simulink model "DCM"  (R2020b)
settings: Solver=ode4  StartTime=0.0  StopTime=SIMULPARAM.T_end  FixedStep=SIMULPARAM.Ts  RelTol=1e-3  EnableMultiTasking=on
undefined symbols (not defined in the file): BAT, C_current, C_speed, CHAS, Chopper, CYCL, DCM, ENV, TRANS
libraries: simulink x1
settings Model: Creator=Huy  LastModifiedBy=mikesimard
settings DataIOCC: SaveFormat=Array  SignalLoggingSaveFormat=ModelDataLogs  SaveOutput=off  SignalLogging=off  SaveTime=off  ReturnWorkspaceOutputs=off
settings OptimizationCC: ExpressionDepthLimit=2147483647  LifeSpan=inf
settings DebuggingCC: AlgebraicLoopMsg=none  SaveWithDisabledLinksMsg=none  UnderspecifiedInitializationDetection=Classic  MergeDetectMultiDrivingBlocksExec=none  MaxConsecutiveZCsMsg=none  SolverPrmCheckMsg=warning  FcnCallInpInsideContextMsg=warning  ModelReferenceDataLoggingMessage=none  ModelReferenceExtraNoncontSigs=none  StateNameClashWarn=warning  SFUnexpectedBacktrackingDiag=warning  SFNoUnconditionalDefaultTransitionDiag=warning  SFExecutionAtInitializationDiag=none  ArithmeticOperatorsInVariantConditions=warning
settings HardwareCC: ProdBitPerPointer=32  ProdBitPerSizeT=32  ProdBitPerPtrDiffT=32  ProdLargestAtomicFloat=None  ProdIntDivRoundTo=Undefined  ProdEndianess=Unspecified  ProdWordSize=32  ProdHWDeviceType=32-bit Generic
settings ModelReferenceCC: PropagateSignalLabelsOutOfModel=off
settings SFSimCC: SimUseLocalCustomCode=off  CustomCodeUndefinedFunction=UseInterfaceOnly
settings RTWCC: RTWUseLocalCustomCode=off
settings CodeAppCC: StateflowObjectComments=on
settings GRTTargetCC: TargetLangStandard=C89/C90 (ANSI)  CombineOutputUpdateFcns=off  GRTInterface=on
settings ConfigComp: CovMetricSettings=dw  CovSaveCumulativeToWorkspaceVar=on  CovSaveSingleToWorkspaceVar=on  CovExternalEMLEnable=off

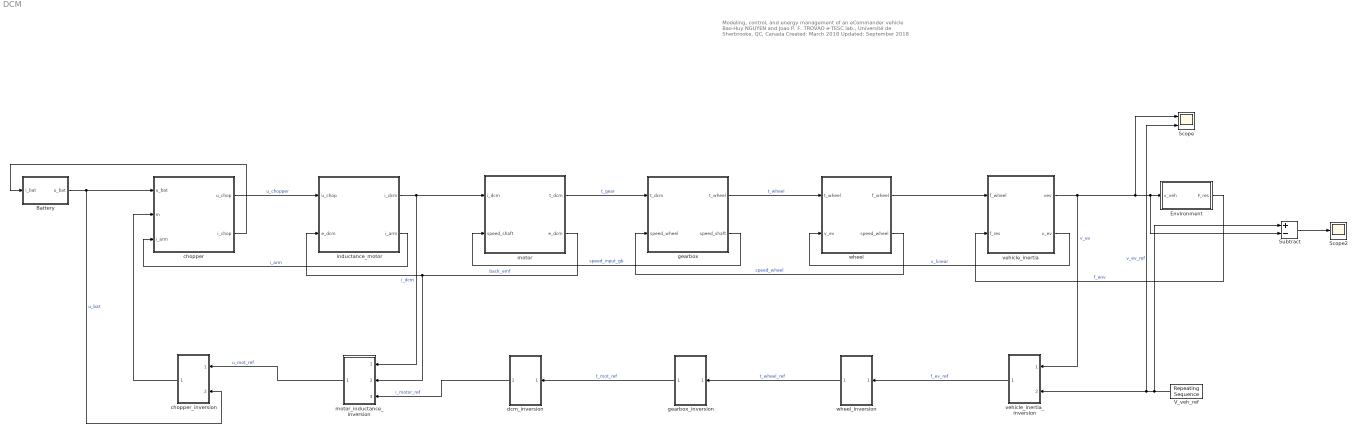
== system DCM ==
  note: Modeling, control, and energy management of an eCommander vehicle
      | Bao-Huy NGUYEN and Joao P. F. TROVAO
      | e-TESC lab., Université de Sherbrooke, QC, Canada
      | Created: March 2018        Updated: September 2018
  Battery : Subsystem  AncestorBlock=simulink/REM/SE
      mask Display:
      | plot(0,0,100,100, 1.2*[50,57.68,60.77,63.08,64.97,66.58,68,69.26,70.4, 	71.42,72.36,78.28,80,78.28,72.36,71.42,70.4, 	69.26,68,66.58,64.97,63.08,60.77,57.68,50,42.32, 	39.23,36.92,35.03,33.42,32,30.74,29.6,28.58, 	27.64,21.72,20,21.72,27.64,28.58,29.6,30.74,32, 	33.42,35.03,36.92,39.23,42.32,50]-10, 1.2*[20,21,22,23,24,25,26,27,28,29,30,40,50,60,70,71,72, 	73,74,75,76,77,78,79,80,79,78,77,76,75,74,73,72, 	71,70,60,50,40,30,29,28,27,26,25,24,23,22,21,20]-10)
      | disp('ES')
  Environment : Subsystem  AncestorBlock=simulink/REM/SE
      mask Display:
      | plot(0,0,100,100, 1.2*[50,57.68,60.77,63.08,64.97,66.58,68,69.26,70.4, 	71.42,72.36,78.28,80,78.28,72.36,71.42,70.4, 	69.26,68,66.58,64.97,63.08,60.77,57.68,50,42.32, 	39.23,36.92,35.03,33.42,32,30.74,29.6,28.58, 	27.64,21.72,20,21.72,27.64,28.58,29.6,30.74,32, 	33.42,35.03,36.92,39.23,42.32,50]-10, 1.2*[20,21,22,23,24,25,26,27,28,29,30,40,50,60,70,71,72, 	73,74,75,76,77,78,79,80,79,78,77,76,75,74,73,72, 	71,70,60,50,40,30,29,28,27,26,25,24,23,22,21,20]-10)
      | disp('MS')
  Scope : Scope  NumInputPorts=2
  Scope2 : Scope
  Subtract : Sum  Inputs=+-
  V_veh_ref : simulink/Sources/Repeating Sequence  rep_seq_t=CYCL.time  rep_seq_y=CYCL.velocity/1.25
  chopper : Subsystem  AncestorBlock=simulink/REM/EA  mask(CM){}
      mask Display: plot(0,0,100,100,[10,10,90,90,10],[90,10,10,90,90])
  chopper_inversion : Subsystem  AncestorBlock=simulink/SMC/Inversion EC avec mesure
      mask Display: plot(0,0,100,100,[10,30,90,70,10],[90,10,10,90,90])
  dcm_inversion : Subsystem  AncestorBlock=simulink/SMC/Inversion EC avec mesure
      mask Display: plot(0,0,100,100,[10,30,90,70,10],[90,10,10,90,90])
  gearbox : Subsystem  AncestorBlock=simulink/REM/EA  mask(CM){}
      mask Display: plot(0,0,100,100,[10,10,90,90,10],[90,10,10,90,90])
  gearbox_inversion : Subsystem  AncestorBlock=simulink/SMC/Inversion EC avec mesure
      mask Display: plot(0,0,100,100,[10,30,90,70,10],[90,10,10,90,90])
  inductance_motor : Subsystem  AncestorBlock=simulink/REM/EA  mask(CM){}
      mask Display: plot(0,0,100,100,[10,10,90,90,10],[90,10,10,90,90], [10,90],[10,90])
  motor : Subsystem  AncestorBlock=simulink/REM/EC EM
      mask Display: plot(0,0,100,100, 1.4*[50,57.68,60.77,63.08,64.97,66.58,68,69.26,70.4, 	71.42,72.36,78.28,80,78.28,72.36,71.42,70.4, 	69.26,68,66.58,64.97,63.08,60.77,57.68,50,42.32, 	39.23,36.92,35.03,33.42,32,30.74,29.6,28.58, 	27.64,21.72,20,21.72,27.64,28.58,29.6,30.74,32, 	33.42,35.03,36.92,39.23,42.32,50]-20, 1.4*[20,21,22,23,24,25,26,27,28,29,30,40,50,60,70,71,72, 	73,74,75,76,77,78,79,80,79,78,77,76,75,74,73,72, 	71,70,60,50,40,30,29,28,27,26,25,24,23,22,21,20]-20)
  motor_inductance_inversion : Subsystem  AncestorBlock=simulink/SMC/Asservissement Correcteur IP
      mask Display: plot(0,0,100,100, [10,30,90,70,10,90],[90,10,10,90,90,10])
  vehicle_inertia : Subsystem  AncestorBlock=simulink/REM/EA  mask(CM){}
      mask Display: plot(0,0,100,100,[10,10,90,90,10],[90,10,10,90,90], [10,90],[10,90])
  vehicle_inertia_inversion : Subsystem  AncestorBlock=simulink/SMC/Asservissement Correcteur IP
      mask Display: plot(0,0,100,100, [10,30,90,70,10,90],[90,10,10,90,90,10])
  wheel : Subsystem  AncestorBlock=simulink/REM/EA  mask(CM){}
      mask Display: plot(0,0,100,100,[10,10,90,90,10],[90,10,10,90,90])
  wheel_inversion : Subsystem  AncestorBlock=simulink/SMC/Inversion EC avec mesure
      mask Display: plot(0,0,100,100,[10,30,90,70,10],[90,10,10,90,90])
  wires:
  chopper_inversion/1(m_chopper) -> chopper/2(m)
  Battery/1(u_bat) -> chopper_inversion/2(u_bat), chopper/1(u_bat)  "u_bat"
  chopper/1(u_chop) -> inductance_motor/1(u_chop)  "u_chopper"
  vehicle_inertia/1(vev) -> Subtract/2, Environment/1(v_veh), Scope/1, vehicle_inertia_inversion/1(v_vehicle)  "v_ev"
  wheel/1(f_wheel) -> vehicle_inertia/1(f_wheel)
  inductance_motor/1(i_dcm) -> motor/1(i_dcm), motor_inductance_inversion/1(i_dcm)  "i_dcm"
  wheel/2(speed_wheel) -> gearbox/2(speed_wheel)  "speed_wheel"
  motor/2(e_dcm) -> inductance_motor/2(e_dcm), motor_inductance_inversion/2(back_emf)  "back_emf"
  motor/1(t_dcm) -> gearbox/1(t_dcm)  "t_gear"
  Environment/1(F_res) -> vehicle_inertia/2(f_res)  "f_env"
  inductance_motor/2(i_arm) -> chopper/3(i_arm)  "i_arm"
  gearbox/1(t_wheel) -> wheel/1(t_wheel)  "t_wheel"
  chopper/2(i_chop) -> Battery/1(i_bat)
  gearbox/2(speed_shaft) -> motor/2(speed_shaft)  "speed_input_gb"
  vehicle_inertia/2(v_ev) -> wheel/2(v_ev)  "v_linear"
  V_veh_ref/1 -> Subtract/1, Scope/2, vehicle_inertia_inversion/2(v_vehicle_ref)  "v_ev_ref"
  vehicle_inertia_inversion/1(f_vehicle_ref) -> wheel_inversion/1(f_vehicle_ref)  "f_ev_ref"
  wheel_inversion/1(t_wheel_ref) -> gearbox_inversion/1(t_wheel_ref)  "t_wheel_ref"
  gearbox_inversion/1(t_motor_ref) -> dcm_inversion/1(t_motor_ref)  "t_mot_ref"
  dcm_inversion/1(i_motor_ref) -> motor_inductance_inversion/3(i_motor_ref)  "i_motor_ref"
  motor_inductance_inversion/1(u_mot_ref) -> chopper_inversion/1(u_mot_ref)  "u_mot_ref"
  Subtract/1 -> Scope2/1

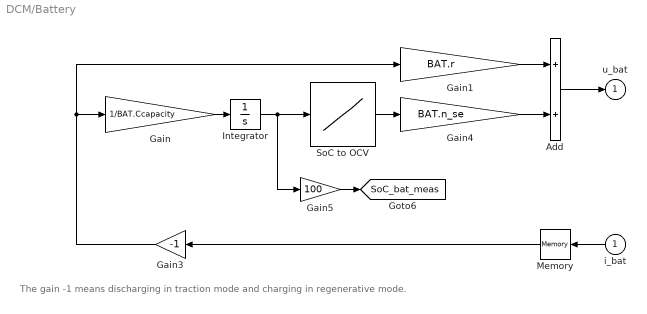
== system DCM/Battery ==
  note: The gain -1 means discharging in traction mode and charging in regenerative mode.
  i_bat : Inport
  Add : Sum
  Gain : Gain  Gain=1/BAT.Ccapacity
  Gain1 : Gain  Gain=BAT.r
  Gain3 : Gain  Gain=-1
  Gain4 : Gain  Gain=BAT.n_se
  Gain5 : Gain  Gain=100
  Integrator : Integrator  InitialCondition=1
  Memory : Memory
  SoC to OCV : Lookup_n-D  NumberOfTableDimensions=1  BreakpointsForDimension1=0.2:0.1:1  Table=11.4:(12-11.4)/((1-0.2)/0.1):12  RndMeth=Simplest  InputSameDT=on
  u_bat : Outport  InitialOutput=0
  tag scope: SoC_bat_meas=global
  wires:
  Integrator/1 -> SoC to OCV/1, Gain5/1
  SoC to OCV/1 -> Gain4/1
  Gain3/1 -> Gain1/1, Gain/1
  Gain5/1 -> [SoC_bat_meas]
  Gain/1 -> Integrator/1
  Gain4/1 -> Add/2
  i_bat/1 -> Memory/1
  Add/1 -> u_bat/1
  Gain1/1 -> Add/1
  Memory/1 -> Gain3/1

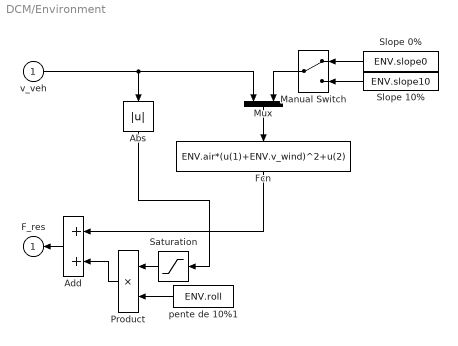
== system DCM/Environment ==
  v_veh : Inport
  Abs : Abs
  Add : Sum
  Fcn : Fcn  Expr=ENV.air*(u(1)+ENV.v_wind)^2+u(2)
  Manual Switch : ManualSwitch
  Mux : Mux  Inputs=2
  Product : Product  RndMeth=Zero
  Saturation : Saturate  UpperLimit=1  LowerLimit=0
  Slope 0% : Constant  Value=ENV.slope0
  Slope 10% : Constant  Value=ENV.slope10
  pente de 10%1 : Constant  Value=ENV.roll
  F_res : Outport  InitialOutput=0
  wires:
  v_veh/1 -> Mux/1, Abs/1
  Mux/1 -> Fcn/1
  Manual Switch/1 -> Mux/2
  Slope 0%/1 -> Manual Switch/1
  Slope 10%/1 -> Manual Switch/2
  Add/1 -> F_res/1
  Fcn/1 -> Add/1
  pente de 10%1/1 -> Product/2
  Product/1 -> Add/2
  Abs/1 -> Saturation/1
  Saturation/1 -> Product/1

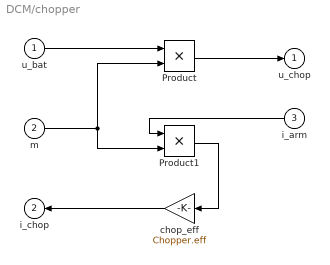
== system DCM/chopper ==
  u_bat : Inport
  m : Inport  Port=2
  i_arm : Inport  Port=3
  Product : Product
  Product1 : Product
  chop_eff : Gain  Gain=Chopper.eff
  u_chop : Outport  InitialOutput=0
  i_chop : Outport  Port=2  InitialOutput=0
  wires:
  u_bat/1 -> Product/1
  Product/1 -> u_chop/1
  chop_eff/1 -> i_chop/1
  Product1/1 -> chop_eff/1
  i_arm/1 -> Product1/1
  m/1 -> Product1/2, Product/2

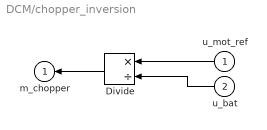
== system DCM/chopper_inversion ==
  u_mot_ref : Inport
  u_bat : Inport  Port=2
  Divide : Product  Inputs=*/
  m_chopper : Outport  InitialOutput=0
  wires:
  Divide/1 -> m_chopper/1
  u_mot_ref/1 -> Divide/1
  u_bat/1 -> Divide/2

== system DCM/dcm_inversion ==
  t_motor_ref : Inport
  1/DCM.phi : Gain  Gain=1/DCM.phi
  i_motor_ref : Outport  InitialOutput=0
  wires:
  t_motor_ref/1 -> 1/DCM.phi/1
  1/DCM.phi/1 -> i_motor_ref/1

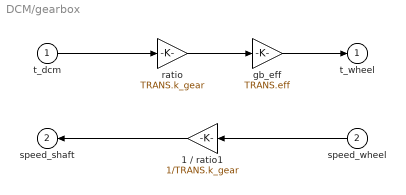
== system DCM/gearbox ==
  t_dcm : Inport
  speed_wheel : Inport  Port=2
  1 / ratio1 : Gain  Gain=1/TRANS.k_gear
  gb_eff : Gain  Gain=TRANS.eff
  ratio : Gain  Gain=TRANS.k_gear
  t_wheel : Outport  InitialOutput=0
  speed_shaft : Outport  Port=2  InitialOutput=0
  wires:
  t_dcm/1 -> ratio/1
  ratio/1 -> gb_eff/1
  gb_eff/1 -> t_wheel/1
  speed_wheel/1 -> 1 / ratio1/1
  1 / ratio1/1 -> speed_shaft/1

== system DCM/gearbox_inversion ==
  t_wheel_ref : Inport
  1 / ratio1 : Gain  Gain=1/TRANS.k_gear
  t_motor_ref : Outport  InitialOutput=0
  wires:
  t_wheel_ref/1 -> 1 / ratio1/1
  1 / ratio1/1 -> t_motor_ref/1

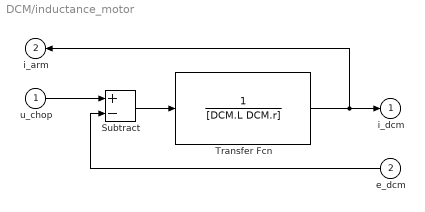
== system DCM/inductance_motor ==
  u_chop : Inport
  e_dcm : Inport  Port=2
  Subtract : Sum  Inputs=+-
  Transfer Fcn : TransferFcn  Denominator=[DCM.L DCM.r]
  i_dcm : Outport  InitialOutput=0
  i_arm : Outport  Port=2  InitialOutput=0
  wires:
  u_chop/1 -> Subtract/1
  e_dcm/1 -> Subtract/2
  Transfer Fcn/1 -> i_arm/1, i_dcm/1
  Subtract/1 -> Transfer Fcn/1

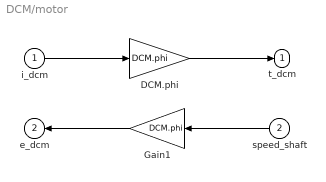
== system DCM/motor ==
  i_dcm : Inport
  speed_shaft : Inport  Port=2
  DCM.phi : Gain  Gain=DCM.phi
  Gain1 : Gain  Gain=DCM.phi
  t_dcm : Outport  InitialOutput=0
  e_dcm : Outport  Port=2  InitialOutput=0
  wires:
  i_dcm/1 -> DCM.phi/1
  DCM.phi/1 -> t_dcm/1
  Gain1/1 -> e_dcm/1
  speed_shaft/1 -> Gain1/1

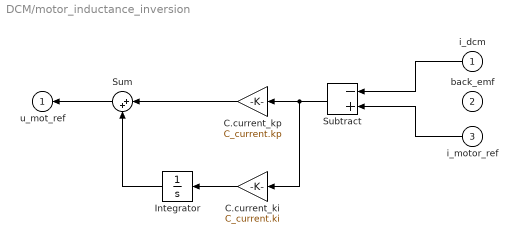
== system DCM/motor_inductance_inversion ==
  i_dcm : Inport
  back_emf : Inport  Port=2
  i_motor_ref : Inport  Port=3
  C.current_ki : Gain  Gain=C_current.ki
  C.current_kp : Gain  Gain=C_current.kp
  Integrator : Integrator
  Subtract : Sum  Inputs=-+
  Sum : Sum  Inputs=|++
  u_mot_ref : Outport  InitialOutput=0
  wires:
  i_motor_ref/1 -> Subtract/2
  i_dcm/1 -> Subtract/1
  Subtract/1 -> C.current_ki/1, C.current_kp/1
  C.current_kp/1 -> Sum/1
  Sum/1 -> u_mot_ref/1
  C.current_ki/1 -> Integrator/1
  Integrator/1 -> Sum/2

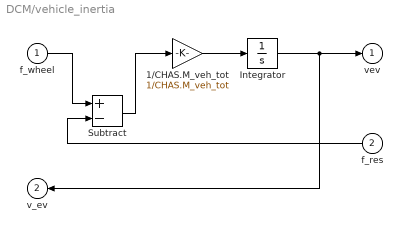
== system DCM/vehicle_inertia ==
  f_wheel : Inport
  f_res : Inport  Port=2
  1/CHAS.M_veh_tot : Gain  Gain=1/CHAS.M_veh_tot
  Integrator : Integrator
  Subtract : Sum  Inputs=+-
  vev : Outport  InitialOutput=0
  v_ev : Outport  Port=2  InitialOutput=0
  wires:
  1/CHAS.M_veh_tot/1 -> Integrator/1
  Integrator/1 -> v_ev/1, vev/1
  f_wheel/1 -> Subtract/1
  f_res/1 -> Subtract/2
  Subtract/1 -> 1/CHAS.M_veh_tot/1

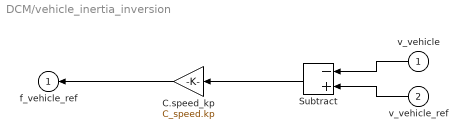
== system DCM/vehicle_inertia_inversion ==
  v_vehicle : Inport
  v_vehicle_ref : Inport  Port=2
  C.speed_kp : Gain  Gain=C_speed.kp
  Subtract : Sum  Inputs=-+
  f_vehicle_ref : Outport  InitialOutput=0
  wires:
  v_vehicle_ref/1 -> Subtract/2
  v_vehicle/1 -> Subtract/1
  Subtract/1 -> C.speed_kp/1
  C.speed_kp/1 -> f_vehicle_ref/1

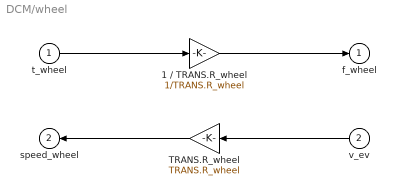
== system DCM/wheel ==
  t_wheel : Inport
  v_ev : Inport  Port=2
  1 / TRANS.R_wheel : Gain  Gain=1/TRANS.R_wheel
  TRANS.R_wheel : Gain  Gain=TRANS.R_wheel
  f_wheel : Outport  InitialOutput=0
  speed_wheel : Outport  Port=2  InitialOutput=0
  wires:
  t_wheel/1 -> 1 / TRANS.R_wheel/1
  1 / TRANS.R_wheel/1 -> f_wheel/1
  v_ev/1 -> TRANS.R_wheel/1
  TRANS.R_wheel/1 -> speed_wheel/1

== system DCM/wheel_inversion ==
  f_vehicle_ref : Inport
  TRANS.R_wheel : Gain  Gain=TRANS.R_wheel
  t_wheel_ref : Outport  InitialOutput=0
  wires:
  f_vehicle_ref/1 -> TRANS.R_wheel/1
  TRANS.R_wheel/1 -> t_wheel_ref/1
